simulink model "FinalEx_with_motion"  (R2020b)
settings: Solver=FixedStepAuto  StartTime=0.0  StopTime=inf  RelTol=1e-3  EnableMultiTasking=on
libraries: arduinomotorcarrierlib x6, eeGeneralControl x2, simulink x1, eePwmGenerator x1, arduinosensorlib x1
settings Model: SimulationMode=external  SILPILModeSetting=veronly  ExtModeTrigDuration=2  Creator=bkhusain  LastModifiedBy=giorg
settings OptimizationCC: EnhancedBackFolding=on  PassReuseOutputArgsAs=Individual arguments  ZeroExternalMemoryAtStartup=off  ZeroInternalMemoryAtStartup=off  MaxStackSize=64  OptimizeBlockOrder=speed  DifferentSizesBufferReuse=on  OptimizationCustomize=off  EfficientTunableParamExpr=on
settings DebuggingCC: ParameterTunabilityLossMsg=error
settings HardwareCC: ProdBitPerPointer=32  ProdBitPerSizeT=32  ProdBitPerPtrDiffT=32  ProdLargestAtomicInteger=Long  ProdLargestAtomicFloat=Double  ProdWordSize=32  ProdHWDeviceType=ARM Compatible->ARM Cortex
settings SFSimCC: MATLABDynamicMemAlloc=off
settings RTWCC: Description=Embedded Coder  SystemTargetFile=ert.tlc  HardwareBoard=Arduino Nano 33 IoT  TemplateMakefile=ert_default_tmf  Toolchain=Arduino ARM  BuildConfiguration=Faster Runs
settings CodeAppCC: ForceParamTrailComments=on  IgnoreCustomStorageClasses=off  OperatorAnnotations=on  SimulinkDataObjDesc=on  SFDataObjDesc=on  InsertBlockDesc=on
settings ERTTargetCC: SupportContinuousTime=on  SupportVariableSizeSignals=on  ExtMode=on  ExtModeStaticAllocSize=8192  ExtModeMexArgs='192.168.137.116' 0 17725

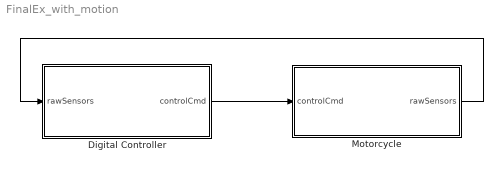
== system FinalEx_with_motion ==
  Digital Controller : Subsystem
      mask Display: image('arduinoNano.png'); % Use "Edit Image" on toolstrip to change.
  Motorcycle : Subsystem
      mask Display: image('motorcycle.jpg'); % Use "Edit Image" on toolstrip to change.
  wires:
  Digital Controller/1(controlCmd) -> Motorcycle/1(controlCmd)
  Motorcycle/1(rawSensors) -> Digital Controller/1(rawSensors)

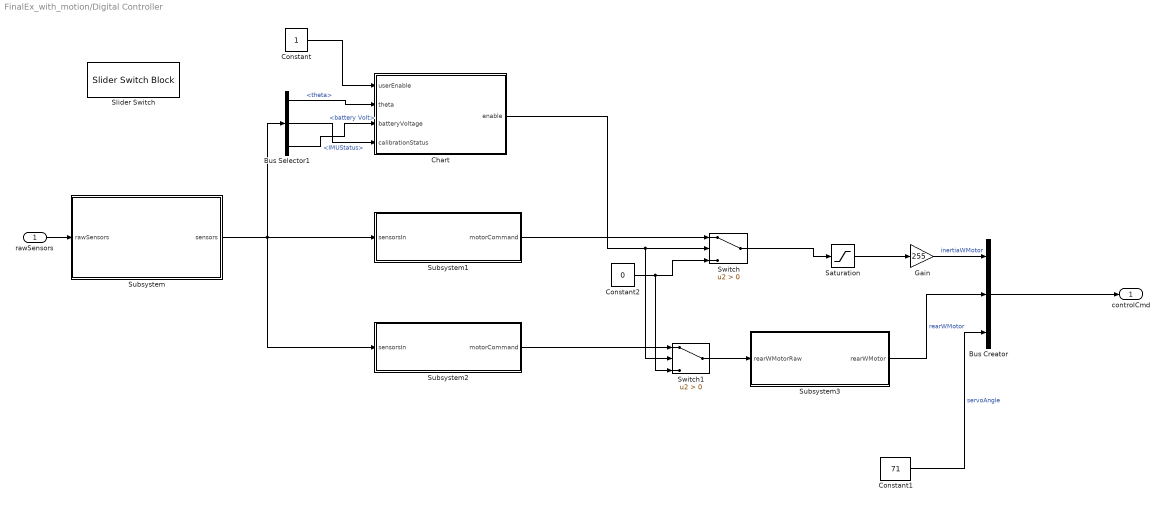
== system FinalEx_with_motion/Digital Controller ==
  rawSensors : Inport
  Bus Creator : BusCreator  Inputs=3
  Bus Selector1 : BusSelector  OutputSignals=theta,IMUStatus,battery Volt
  Chart : Stateflow chart  TreatAsAtomicUnit=on
  Constant : Constant
  Constant1 : Constant  Value=71  SampleTime=0.01
  Constant2 : Constant  Value=0  SampleTime=0.01
  Gain : Gain  Gain=255
  Saturation : Saturate  UpperLimit=1  LowerLimit=-1
  Slider Switch : SliderSwitchBlock
      settings: Values={{'Off', 'On'}, [0 1]}
  Subsystem : Subsystem
  Subsystem1 : Subsystem
  Subsystem2 : Subsystem
  Subsystem3 : Subsystem
  Switch : Switch  Criteria=u2 > Threshold
  Switch1 : Switch  Criteria=u2 > Threshold
  controlCmd : Outport
  wires:
  Bus Creator/1 -> controlCmd/1
  Switch/1 -> Saturation/1
  rawSensors/1 -> Subsystem/1(rawSensors)
  Subsystem/1(sensors) -> Subsystem2/1(sensorsIn), Subsystem1/1(sensorsIn), Bus Selector1/1
  Constant/1 -> Chart/1(userEnable)
  Bus Selector1/1 -> Chart/2(theta)  "<theta>"
  Bus Selector1/2 -> Chart/4(calibrationStatus)  "<IMUStatus>"
  Bus Selector1/3 -> Chart/3(batteryVoltage)  "<battery Volt>"
  Subsystem1/1(motorCommand) -> Switch/1
  Constant2/1 -> Switch1/3, Switch/3
  Chart/1(enable) -> Switch1/2, Switch/2
  Switch1/1 -> Subsystem3/1(rearWMotorRaw)
  Subsystem2/1(motorCommand) -> Switch1/1
  Constant1/1 -> Bus Creator/3  "servoAngle"
  Saturation/1 -> Gain/1
  Gain/1 -> Bus Creator/1  "inertiaWMotor"
  Subsystem3/1(rearWMotor) -> Bus Creator/2  "rearWMotor"

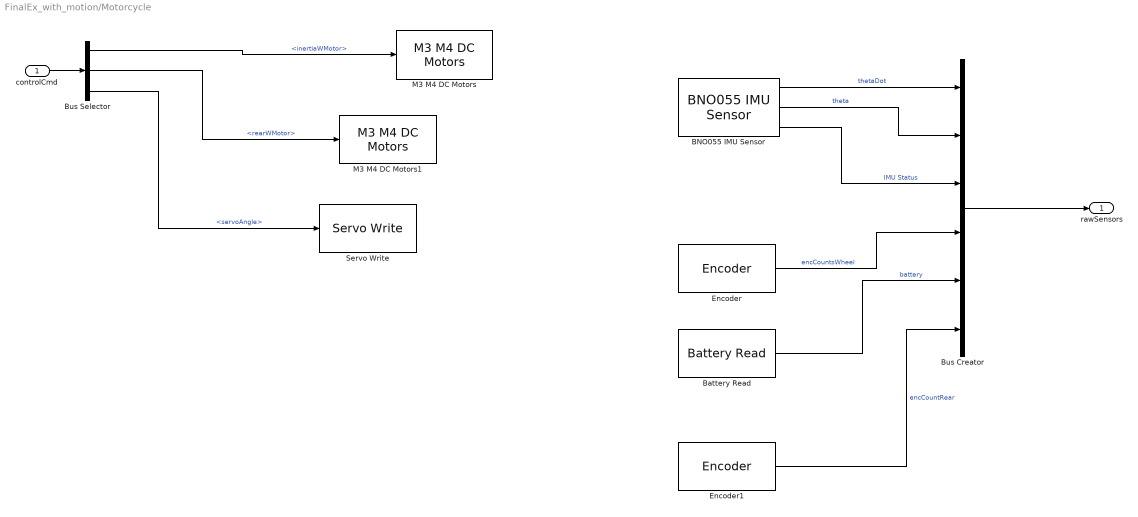
== system FinalEx_with_motion/Motorcycle ==
  controlCmd : Inport
  BNO055 IMU Sensor : arduinosensorlib/BNO055 IMU Sensor  SlaveAddress=0x28  OperationMode=Fusion  Accel=off  AngularRate=on  MagField=off  EulerAngles=on  Quat=off  LinearAccel=off  GravityVector=off  AccelRange=4G  AccelBW=62.5 Hz  GyroRange=2000 dps  GyroBW=32 Hz  MagODR=10 Hz  SampleTime=0.01  blockPlatform=ARDUINO
      settings: SourceProductBaseCode=ARDUINO
  Battery Read : arduinomotorcarrierlib/Battery Read  SlaveAddress=uint8( hex2dec( '66' ) )  blockPlatform=ARDUINO  SampleTime=0.01
      settings: SourceProductBaseCode=ARDUINO
  Bus Creator : BusCreator  Inputs=6
  Bus Selector : BusSelector  OutputSignals=inertiaWMotor,rearWMotor,servoAngle
  Encoder : arduinomotorcarrierlib/Encoder  SlaveAddress=uint8( hex2dec( '66' ) )  blockPlatform=ARDUINO  Encoder=1  ShowSpeed=off  ResetOption=on  SampleTime=0.01
      settings: SourceProductBaseCode=ARDUINO
  Encoder1 : arduinomotorcarrierlib/Encoder  SlaveAddress=uint8( hex2dec( '66' ) )  blockPlatform=ARDUINO  Encoder=2  ShowSpeed=off  ResetOption=on  SampleTime=0.01
      settings: SourceProductBaseCode=ARDUINO
  M3 M4 DC Motors : arduinomotorcarrierlib/M3 M4 DC Motors  MotorNumber=M3  forwardPinNumber=3  reversePinNumber=2
      settings: SourceProductBaseCode=ARDUINO
  M3 M4 DC Motors1 : arduinomotorcarrierlib/M3 M4 DC Motors  MotorNumber=M4  forwardPinNumber=4  reversePinNumber=5
      settings: SourceProductBaseCode=ARDUINO
  Servo Write : arduinomotorcarrierlib/Servo Write  SlaveAddress=uint8( hex2dec( '66' ) )  blockPlatform=ARDUINO  MotorNumber=3  MotorCarrierPWMFreq=100
      settings: SourceProductBaseCode=ARDUINO
  rawSensors : Outport
  wires:
  BNO055 IMU Sensor/1 -> Bus Creator/1  "thetaDot"
  BNO055 IMU Sensor/2 -> Bus Creator/2  "theta"
  BNO055 IMU Sensor/3 -> Bus Creator/3  "IMU Status"
  Encoder/1 -> Bus Creator/4  "encCountsWheel"
  Battery Read/1 -> Bus Creator/5  "battery"
  Bus Creator/1 -> rawSensors/1
  controlCmd/1 -> Bus Selector/1
  Bus Selector/1 -> M3 M4 DC Motors/1  "<inertiaWMotor>"
  Encoder1/1 -> Bus Creator/6  "encCountRear"
  Bus Selector/3 -> Servo Write/1  "<servoAngle>"
  Bus Selector/2 -> M3 M4 DC Motors1/1  "<rearWMotor>"

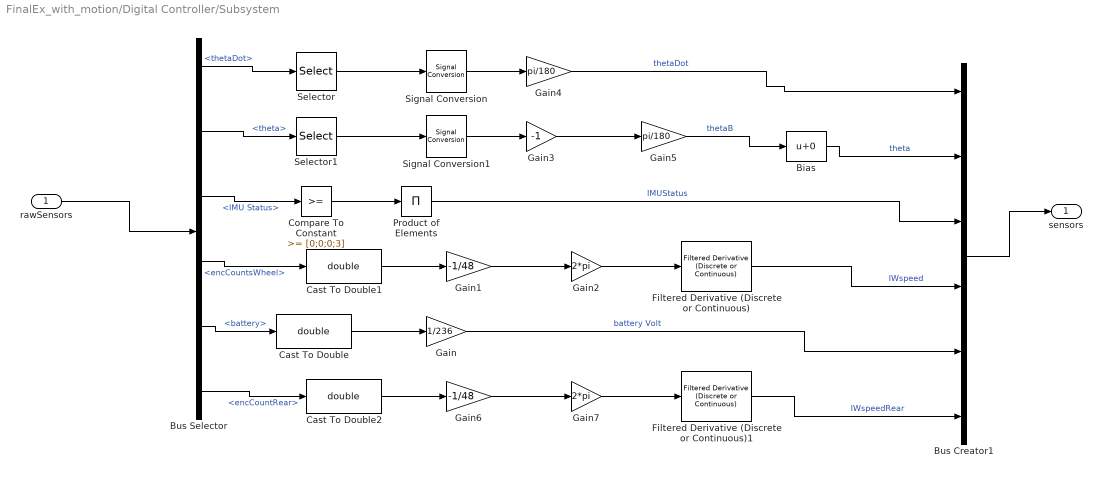
== system FinalEx_with_motion/Digital Controller/Subsystem ==
  rawSensors : Inport
  Bias : Bias
  Bus Creator1 : BusCreator  Inputs=6
  Bus Selector : BusSelector  OutputSignals=thetaDot,theta,IMU Status,encCountsWheel,battery,encCountRear
  Cast To Double : DataTypeConversion  OutDataTypeStr=double
  Cast To Double1 : DataTypeConversion  OutDataTypeStr=double
  Cast To Double2 : DataTypeConversion  OutDataTypeStr=double
  Compare To Constant : simulink/Logic and Bit Operations/Compare To Constant  relop=>=  const=[0;0;0;3]  OutDataTypeStr=boolean
  Filtered Derivative (Discrete or Continuous) : eeGeneralControl/Filtered Derivative (Discrete or Continuous)  K=1  T=0.1  B=inf  A=-inf  minRatio=10  init_option=Inherited from block input  x0=0  Ts=0.01
      settings: SourceProductBaseCode=PS
  Filtered Derivative (Discrete or Continuous)1 : eeGeneralControl/Filtered Derivative (Discrete or Continuous)  K=1  T=0.1  B=inf  A=-inf  minRatio=10  init_option=Inherited from block input  x0=0  Ts=0.01
      settings: SourceProductBaseCode=PS
  Gain : Gain  Gain=1/236
  Gain1 : Gain  Gain=-1/48
  Gain2 : Gain  Gain=2*pi
  Gain3 : Gain  Gain=-1
  Gain4 : Gain  Gain=pi/180
  Gain5 : Gain  Gain=pi/180
  Gain6 : Gain  Gain=-1/48
  Gain7 : Gain  Gain=2*pi
  Product of Elements : Product  Inputs=*
  Selector : Selector  InputPortWidth=3  IndexOptions=Index vector (dialog)  Indices=[2]  OutputSizes=1
  Selector1 : Selector  InputPortWidth=3  IndexOptions=Index vector (dialog)  Indices=[2]  OutputSizes=1
  Signal Conversion : SignalConversion  OverrideOpt=off
  Signal Conversion1 : SignalConversion  OverrideOpt=off
  sensors : Outport
  wires:
  Signal Conversion1/1 -> Gain3/1
  Product of Elements/1 -> Bus Creator1/3  "IMUStatus"
  Bus Selector/1 -> Selector/1  "<thetaDot>"
  Selector1/1 -> Signal Conversion1/1
  Gain1/1 -> Gain2/1
  Bus Selector/3 -> Compare To Constant/1  "<IMU Status>"
  Bus Creator1/1 -> sensors/1
  rawSensors/1 -> Bus Selector/1
  Cast To Double1/1 -> Gain1/1
  Selector/1 -> Signal Conversion/1
  Gain5/1 -> Bias/1  "thetaB"
  Filtered Derivative (Discrete or Continuous)/1 -> Bus Creator1/4  "IWspeed"
  Gain3/1 -> Gain5/1
  Bus Selector/2 -> Selector1/1  "<theta>"
  Bus Selector/4 -> Cast To Double1/1  "<encCountsWheel>"
  Cast To Double/1 -> Gain/1
  Bus Selector/5 -> Cast To Double/1  "<battery>"
  Gain/1 -> Bus Creator1/5  "battery Volt"
  Gain2/1 -> Filtered Derivative (Discrete or Continuous)/1
  Signal Conversion/1 -> Gain4/1
  Compare To Constant/1 -> Product of Elements/1
  Gain4/1 -> Bus Creator1/1  "thetaDot"
  Bias/1 -> Bus Creator1/2  "theta"
  Bus Selector/6 -> Cast To Double2/1  "<encCountRear>"
  Cast To Double2/1 -> Gain6/1
  Gain6/1 -> Gain7/1
  Gain7/1 -> Filtered Derivative (Discrete or Continuous)1/1
  Filtered Derivative (Discrete or Continuous)1/1 -> Bus Creator1/6  "IWspeedRear"

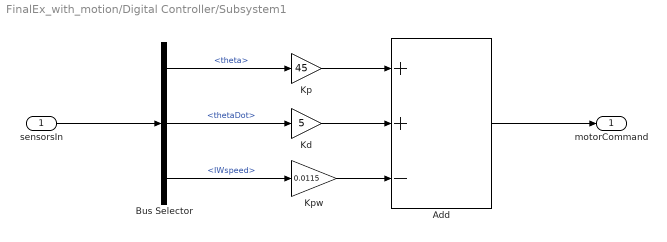
== system FinalEx_with_motion/Digital Controller/Subsystem1 ==
  sensorsIn : Inport
  Add : Sum  Inputs=++-
  Bus Selector : BusSelector  OutputSignals=theta,thetaDot,IWspeed
  Kd : Gain  Gain=5
  Kp : Gain  Gain=45
  Kpw : Gain  Gain=0.0115
  motorCommand : Outport
  wires:
  sensorsIn/1 -> Bus Selector/1
  Add/1 -> motorCommand/1
  Kpw/1 -> Add/3
  Kd/1 -> Add/2
  Kp/1 -> Add/1
  Bus Selector/1 -> Kp/1  "<theta>"
  Bus Selector/2 -> Kd/1  "<thetaDot>"
  Bus Selector/3 -> Kpw/1  "<IWspeed>"

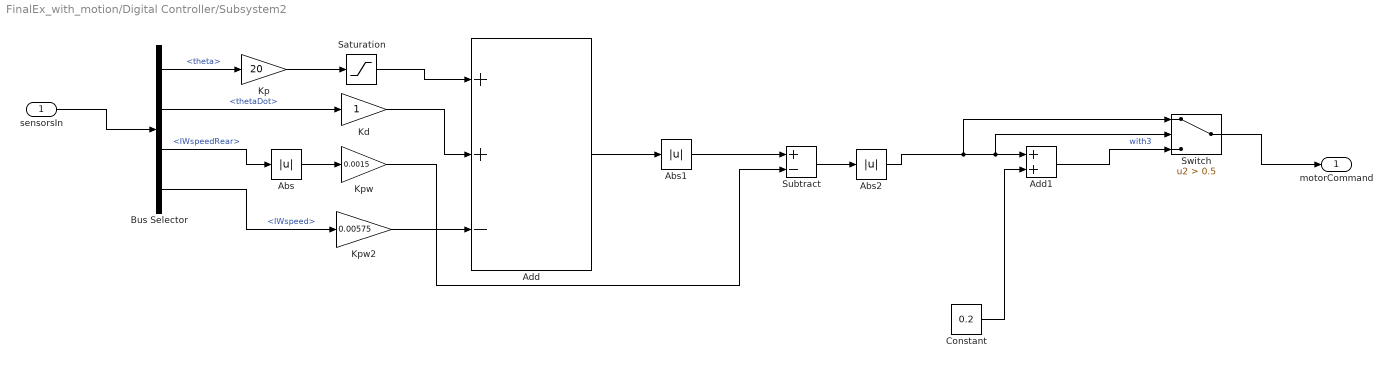
== system FinalEx_with_motion/Digital Controller/Subsystem2 ==
  sensorsIn : Inport
  Abs : Abs
  Abs1 : Abs
  Abs2 : Abs
  Add : Sum  Inputs=++-
  Add1 : Sum
  Bus Selector : BusSelector  OutputSignals=theta,thetaDot,IWspeedRear,IWspeed
  Constant : Constant  Value=0.2  SampleTime=0.01
  Kd : Gain
  Kp : Gain  Gain=20
  Kpw : Gain  Gain=0.0015
  Kpw2 : Gain  Gain=0.00575
  Saturation : Saturate  UpperLimit=3  LowerLimit=-3
  Subtract : Sum  Inputs=+-
  Switch : Switch  Criteria=u2 > Threshold  Threshold=0.5
  motorCommand : Outport
  wires:
  sensorsIn/1 -> Bus Selector/1
  Add/1 -> Abs1/1
  Kpw/1 -> Subtract/2
  Kd/1 -> Add/2
  Bus Selector/1 -> Kp/1  "<theta>"
  Bus Selector/2 -> Kd/1  "<thetaDot>"
  Bus Selector/3 -> Abs/1  "<IWspeedRear>"
  Kpw2/1 -> Add/3
  Bus Selector/4 -> Kpw2/1  "<IWspeed>"
  Abs/1 -> Kpw/1
  Kp/1 -> Saturation/1
  Saturation/1 -> Add/1
  Abs1/1 -> Subtract/1
  Constant/1 -> Add1/2
  Add1/1 -> Switch/3  "with3"
  Subtract/1 -> Abs2/1
  Abs2/1 -> Switch/1, Switch/2, Add1/1
  Switch/1 -> motorCommand/1

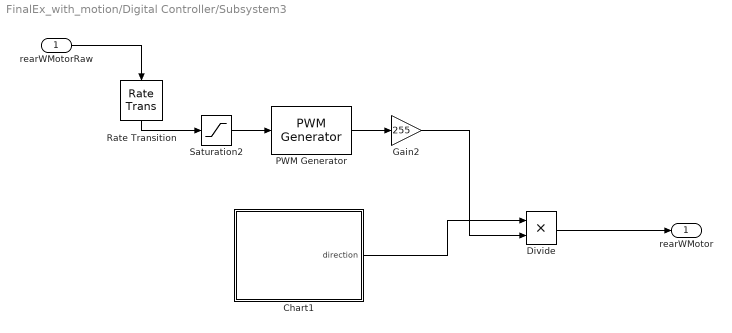
== system FinalEx_with_motion/Digital Controller/Subsystem3 ==
  rearWMotorRaw : Inport
  Chart1 : Stateflow chart  TreatAsAtomicUnit=on
  Divide : Product  Inputs=**
  Gain2 : Gain  Gain=255
  PWM Generator : eePwmGenerator/PWM Generator  CarrCount=Up  Tper=0.05  Ts=0.005
  Rate Transition : RateTransition
  Saturation2 : Saturate  UpperLimit=1  LowerLimit=0
  rearWMotor : Outport
  wires:
  Rate Transition/1 -> Saturation2/1
  Saturation2/1 -> PWM Generator/1
  Divide/1 -> rearWMotor/1
  Gain2/1 -> Divide/2
  Chart1/1(direction) -> Divide/1
  PWM Generator/1 -> Gain2/1
  rearWMotorRaw/1 -> Rate Transition/1

== stateflow chart FinalEx_with_motion/Digital Controller/Subsystem3/Chart1 ==
  state out8
    entry: direction = 1;
  state out5
    entry: direction = 0;
  state out7
    entry: direction = 0;
  state out6
    entry: direction = -1;
  (default) -> out5
  out8 -> out5 : [after(5,sec)]
  out7 -> out8 : [after(3,sec)]
  out5 -> out6 : [after(3,sec)]
  out6 -> out7 : [after(5,sec)]
  data: direction output

== stateflow chart FinalEx_with_motion/Digital Controller/Chart ==
  state checkFallen [parallel]
    settings: executionOrder=1
    state Fallen
      entry: upright = false;
    state Standing
      entry: upright = true;
    (default) -> Fallen
    Fallen -> Standing : [abs(theta)<pi*12/180]
    Standing -> Fallen : [abs(theta) > pi*12/180]
  state checkIMUCalib [parallel]
    settings: executionOrder=2
    state imuNotCalibrated
      entry:
      IMUCalibrated = false;
    state imuCalibrated
      entry:
      IMUCalibrated = true;
    (default) -> imuNotCalibrated
    imuNotCalibrated -> imuCalibrated : [calibrationStatus == true]
  state checkBattery [parallel]
    settings: executionOrder=3
    state batteryNotCharged
      entry:
      batteryOK = false;
    state batteryCharged
      entry:
      batteryOK = true;
    (default) -> batteryNotCharged
    batteryNotCharged -> batteryCharged : [batteryVoltage > 3]
    batteryCharged -> batteryNotCharged : [batteryVoltage <= 3]
  state calculateEnable [parallel]
    settings: executionOrder=4
    state disableControl
      entry:
      enable = false
    state enableControl
      entry:
      enable = true
    (default) -> disableControl
    disableControl -> enableControl : [userEnable && batteryOK && IMUCalibrated && upright]
    enableControl -> disableControl : [not(userEnable) || not(batteryOK) || not(IMUCalibrated) || not(upright)]
  data: userEnable input; theta input; enable output; upright local; IMUCalibrated local; batteryOK local; batteryVoltage input; calibrationStatus input
